simulink model "NeuromuscularModel"  (R2019b)
settings: Solver=ode15s  StartTime=0.0  StopTime=30  MaxStep=.01  RelTol=1e-4  AbsTol=1e-6  EnableMultiTasking=on
values from neighbouring files (symbols this model uses):
  legLengthClr = 0.85    [ControlParams.m]    (also in assignGains.m = Gains(20); assignGainsSagittal.m = GainsSagittal(39))
  LongDelay = 0.020/2    (= 0.01)    [ControlParams.m]
  MidDelay = 0.010/2    (= 0.005)    [ControlParams.m]
  N = {S.name}    [mergeCompareEnergyCosts.m]
  ShortDelay = 0.005/2    (= 0.0025)    [ControlParams.m]
  simbiconGainD = 5*pi/180    (= 0.0872664625997)    [ControlParams.m]    (also in assignGains.m = Gains(21); assignGainsSagittal.m = GainsSagittal(41))
  simbiconGainV = 5*pi/180    (= 0.0872664625997)    [ControlParams.m]    (also in assignGains.m = Gains(22); assignGainsSagittal.m = GainsSagittal(42))
  simbiconLegAngle0 = 70*pi/180    (= 1.2217304764)    [ControlParams.m]    (also in assignGains.m = Gains(23); assignGainsSagittal.m = GainsSagittal(40))
  X = ~cellfun('isempty',strfind(N,'compareEnergyCost'))    [mergeCompareEnergyCosts.m]
undefined symbols (not defined in the file or in its folder): footCenterToCGDist, footInertia, footMass, g, LceOffsetTA, loptGAS, loptTA, lslackGAS, phimaxGASa, phimaxGASk, phirefGASa, phirefGASk, rGASa, rGASk, rhoGASa, rhoGASk, Y, Z
libraries: NeuroMuscularLibrary x85, nesl_utility x23, sm_lib x16, simulink x4, simulink_extras x2
(part 2 of 2)

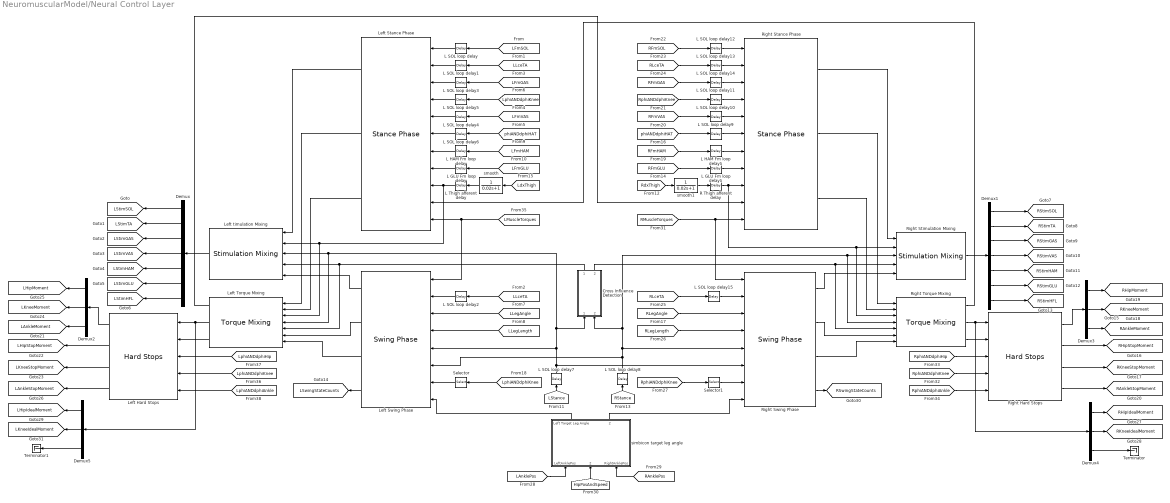
== system NeuromuscularModel/Neural Control Layer ==
  Cross Influence Detection : Subsystem
  Demux : Demux  Outputs=7
  Demux1 : Demux  Outputs=7
  Demux{2..5} (4 alike) : Demux  Outputs=3
  L GLU Fm loop delay : TransportDelay  DelayTime=ShortDelay
  L GLU Fm loop delay1 : TransportDelay  DelayTime=ShortDelay
  L HAM Fm loop delay : TransportDelay  DelayTime=ShortDelay
  L HAM Fm loop delay1 : TransportDelay  DelayTime=ShortDelay
  L SOL loop delay{,1..3,12..15} (8 alike) : TransportDelay  DelayTime=LongDelay
  L SOL loop delay{4..5,7..8,10..11} (6 alike) : TransportDelay  DelayTime=MidDelay
  L SOL loop delay6 : TransportDelay  DelayTime=ShortDelay
  L SOL loop delay9 : TransportDelay  DelayTime=ShortDelay
  L Thigh afferent delay : TransportDelay  DelayTime=ShortDelay
  Left Hard Stops : NeuroMuscularLibrary/Hard Stops  SystemSampleTime=-1  Latency=0  AutoFrameSizeCalculation=off
  Left Stance Phase : NeuroMuscularLibrary/Stance Phase  GainHAM=GainHAM  GainGLU=GainGLU  GainSOL=GainSOL  GainSOLTA=GainSOLTA  GainTA=GainTA  GainGAS=GainGAS  GainVAS=GainVAS  GainKneeOverExt=GainKneeOverExt  PosGainGG=PosGainGG  SpeedGainGG=SpeedGainGG  Kglu=Kglu
  Left Swing Phase : NeuroMuscularLibrary/Swing Phase  GainTA=GainTA  hipPGain=hipPGain  hipDGain=hipDGain  legAngleFilter=legAngleFilter  kneeFlexGain=kneeFlexGain  kneeHoldGain1=kneeHoldGain1  kneeHoldGain2=kneeHoldGain2  kneeStopGain=kneeStopGain  kneeExtendGain=kneeExtendGain  legLengthClr=legLengthClr
  Left Torque Mixing : NeuroMuscularLibrary/Torque Mixing  SystemSampleTime=-1  Latency=0  AutoFrameSizeCalculation=off
  Left timulation Mixing : NeuroMuscularLibrary/Stimulation Mixing  SystemSampleTime=-1  Latency=0  AutoFrameSizeCalculation=off
  R Thigh afferent delay : TransportDelay  DelayTime=ShortDelay
  Right Hard Stops : NeuroMuscularLibrary/Hard Stops  SystemSampleTime=-1  Latency=0  AutoFrameSizeCalculation=off
  Right Stance Phase : NeuroMuscularLibrary/Stance Phase  GainHAM=GainHAM  GainGLU=GainGLU  GainSOL=GainSOL  GainSOLTA=GainSOLTA  GainTA=GainTA  GainGAS=GainGAS  GainVAS=GainVAS  GainKneeOverExt=GainKneeOverExt  PosGainGG=PosGainGG  SpeedGainGG=SpeedGainGG  Kglu=Kglu
  Right Stimulation Mixing : NeuroMuscularLibrary/Stimulation Mixing  SystemSampleTime=-1  Latency=0  AutoFrameSizeCalculation=off
  Right Swing Phase : NeuroMuscularLibrary/Swing Phase  GainTA=GainTA  hipPGain=hipPGain  hipDGain=hipDGain  legAngleFilter=legAngleFilter  kneeFlexGain=kneeFlexGain  kneeHoldGain1=kneeHoldGain1  kneeHoldGain2=kneeHoldGain2  kneeStopGain=kneeStopGain  kneeExtendGain=kneeExtendGain  legLengthClr=legLengthClr
  Right Torque Mixing : NeuroMuscularLibrary/Torque Mixing  SystemSampleTime=-1  Latency=0  AutoFrameSizeCalculation=off
  Selector : Selector  InputPortWidth=2  IndexOptions=Index vector (dialog)  Indices=2  OutputSizes=1
  Selector1 : Selector  InputPortWidth=2  IndexOptions=Index vector (dialog)  Indices=2  OutputSizes=1
  Terminator : Terminator
  Terminator1 : Terminator
  simbicon target leg angle : Subsystem
  smooth : TransferFcn  Denominator=[0.02 1]
  smooth1 : TransferFcn  Denominator=[0.02 1]
  tag scope: LAnkleMoment=global, LAnkleStopMoment=global, LHipIdealMoment=global, LHipMoment=global, LHipStopMoment=global, LKneeIdealMoment=global, LKneeMoment=global, LKneeStopMoment=global, LStimGAS=global, LStimGLU=global, LStimHAM=global, LStimHFL=global, LStimSOL=global, LStimTA=global, LStimVAS=global, LSwingStateCounts=global, RAnkleMoment=global, RAnkleStopMoment=global, RHipIdealMoment=global, RHipMoment=global, RHipStopMoment=global, RKneeIdealMoment=global, RKneeMoment=global, RKneeStopMoment=global, RStimGAS=global, RStimGLU=global, RStimHAM=global, RStimHFL=global, RStimSOL=global, RStimTA=global, RStimVAS=global, RSwingStateCounts=global
  wires:
  [LFmSOL] -> L SOL loop delay/1
  L SOL loop delay/1 -> Left Stance Phase/1
  [LLceTA] -> L SOL loop delay1/1
  L SOL loop delay1/1 -> Left Stance Phase/2
  Demux/1 -> [LStimSOL]
  Demux/2 -> [LStimTA]
  Demux/3 -> [LStimGAS]
  [LFmGAS] -> L SOL loop delay3/1
  L SOL loop delay3/1 -> Left Stance Phase/3
  [LLceTA] -> L SOL loop delay2/1
  L SOL loop delay4/1 -> Left Stance Phase/5
  [LFmVAS] -> L SOL loop delay4/1
  L SOL loop delay5/1 -> Left Stance Phase/4
  [LphiANDdphiKnee] -> L SOL loop delay5/1
  Demux/4 -> [LStimVAS]
  [phiANDdphiHAT] -> L SOL loop delay6/1
  L SOL loop delay6/1 -> Left Stance Phase/6
  Demux/5 -> [LStimHAM]
  Demux/6 -> [LStimGLU]
  Demux/7 -> [LStimHFL]
  [LdxThigh] -> smooth/1
  smooth/1 -> L Thigh afferent delay/1
  [RdxThigh] -> smooth1/1
  smooth1/1 -> R Thigh afferent delay/1
  [LFmHAM] -> L HAM Fm loop delay/1
  [LFmGLU] -> L GLU Fm loop delay/1
  L SOL loop delay7/1 -> Left Torque Mixing/4, Left timulation Mixing/3, Cross Influence Detection/1(LStance), Left Swing Phase/5, Right Swing Phase/6
  [RFmHAM] -> L HAM Fm loop delay1/1
  [RFmGLU] -> L GLU Fm loop delay1/1
  [phiANDdphiHAT] -> L SOL loop delay9/1
  L SOL loop delay9/1 -> Right Stance Phase/6
  Demux1/1 -> [RStimSOL]
  Demux1/2 -> [RStimTA]
  Demux1/4 -> [RStimVAS]
  Demux1/5 -> [RStimHAM]
  Demux1/7 -> [RStimHFL]
  Demux1/3 -> [RStimGAS]
  [LStance] -> L SOL loop delay7/1
  [RStance] -> L SOL loop delay8/1
  [RFmVAS] -> L SOL loop delay10/1
  [RphiANDdphiKnee] -> L SOL loop delay11/1
  L SOL loop delay10/1 -> Right Stance Phase/5
  L SOL loop delay11/1 -> Right Stance Phase/4
  L SOL loop delay12/1 -> Right Stance Phase/1
  [RFmSOL] -> L SOL loop delay12/1
  [RLceTA] -> L SOL loop delay13/1
  L SOL loop delay13/1 -> Right Stance Phase/2
  [RFmGAS] -> L SOL loop delay14/1
  L SOL loop delay14/1 -> Right Stance Phase/3
  [RLceTA] -> L SOL loop delay15/1
  Demux1/6 -> [RStimGLU]
  L Thigh afferent delay/1 -> Left Torque Mixing/3, Left timulation Mixing/2, Left Stance Phase/9
  L HAM Fm loop delay/1 -> Left Stance Phase/7
  L GLU Fm loop delay/1 -> Left Stance Phase/8
  R Thigh afferent delay/1 -> Right Stimulation Mixing/2, Right Torque Mixing/3, Right Stance Phase/9
  L HAM Fm loop delay1/1 -> Right Stance Phase/7
  L GLU Fm loop delay1/1 -> Right Stance Phase/8
  L SOL loop delay15/1 -> Right Swing Phase/2
  L SOL loop delay2/1 -> Left Swing Phase/2
  Right Stimulation Mixing/1 -> Demux1/1
  Right Stance Phase/1 -> Right Stimulation Mixing/1
  L SOL loop delay8/1 -> Right Stimulation Mixing/3, Right Torque Mixing/4, Cross Influence Detection/2(RStance), Right Swing Phase/5, Left Swing Phase/6
  Cross Influence Detection/2(LeftLeading) -> Right Stimulation Mixing/4, Right Torque Mixing/5
  Left timulation Mixing/1 -> Demux/1
  Left Stance Phase/1 -> Left timulation Mixing/1
  Cross Influence Detection/1(RightLeading) -> Left Torque Mixing/5, Left timulation Mixing/4
  Demux3/1 -> [RHipMoment]
  Demux3/2 -> [RKneeMoment]
  [LLegAngle] -> Left Swing Phase/3
  [LLegLength] -> Left Swing Phase/4
  [RLegAngle] -> Right Swing Phase/3
  [RLegLength] -> Right Swing Phase/4
  [RphiANDdphiKnee] -> Selector1/1
  Selector1/1 -> Right Swing Phase/7
  [LAnklePos] -> simbicon target leg angle/1(LeftAnklePos)
  [RAnklePos] -> simbicon target leg angle/3(RightAnklePos)
  Right Swing Phase/1 -> Right Stimulation Mixing/5
  [LphiANDdphiKnee] -> Selector/1
  Selector/1 -> Left Swing Phase/7
  Left Swing Phase/1 -> Left timulation Mixing/5
  [HipPosAndSpeed] -> simbicon target leg angle/2(HIPposAndSpeed)
  simbicon target leg angle/2(Right Target Leg Angle) -> Right Swing Phase/8
  simbicon target leg angle/1(Left Target Leg Angle) -> Left Swing Phase/8
  Right Swing Phase/4 -> [RSwingStateCounts]
  Left Swing Phase/4 -> [LSwingStateCounts]
  Demux3/3 -> [RAnkleMoment]
  [RphiANDdphiKnee] -> Right Hard Stops/4
  [RphiANDdphiHip] -> Right Hard Stops/3
  [RphiANDdphiAnkle] -> Right Hard Stops/5
  Right Hard Stops/2 -> [RHipStopMoment]
  Right Hard Stops/3 -> [RKneeStopMoment]
  Right Hard Stops/4 -> [RAnkleStopMoment]
  [LMuscleTorques] -> Left Swing Phase/1, Left Stance Phase/11
  Demux2/1 -> [LHipMoment]
  Demux2/3 -> [LAnkleMoment]
  Left Hard Stops/1 -> Demux2/1
  [LphiANDdphiKnee] -> Left Hard Stops/4
  [LphiANDdphiHip] -> Left Hard Stops/3
  Left Hard Stops/2 -> [LHipStopMoment]
  Left Hard Stops/3 -> [LKneeStopMoment]
  Left Hard Stops/4 -> [LAnkleStopMoment]
  Left Stance Phase/2 -> Left Torque Mixing/1
  Demux2/2 -> [LKneeMoment]
  Right Torque Mixing/2 -> Demux4/1, Right Hard Stops/1
  Right Hard Stops/1 -> Demux3/1
  [RMuscleTorques] -> Right Swing Phase/1, Right Stance Phase/11
  Demux4/1 -> [RHipIdealMoment]
  Demux4/2 -> [RKneeIdealMoment]
  Demux4/3 -> Terminator/1
  Right Swing Phase/3 -> Right Torque Mixing/7
  Right Swing Phase/2 -> Right Torque Mixing/6
  Right Stance Phase/3 -> Right Torque Mixing/2
  Right Stance Phase/2 -> Right Torque Mixing/1
  Right Torque Mixing/3 -> Right Hard Stops/2
  Right Torque Mixing/1 -> Left Stance Phase/10
  [LphiANDdphiAnkle] -> Left Hard Stops/5
  Left Torque Mixing/2 -> Demux5/1, Left Hard Stops/1
  Left Torque Mixing/3 -> Left Hard Stops/2
  Left Torque Mixing/1 -> Right Stance Phase/10
  Left Stance Phase/3 -> Left Torque Mixing/2
  Left Swing Phase/2 -> Left Torque Mixing/6
  Left Swing Phase/3 -> Left Torque Mixing/7
  Demux5/1 -> [LHipIdealMoment]
  Demux5/2 -> [LKneeIdealMoment]
  Demux5/3 -> Terminator1/1

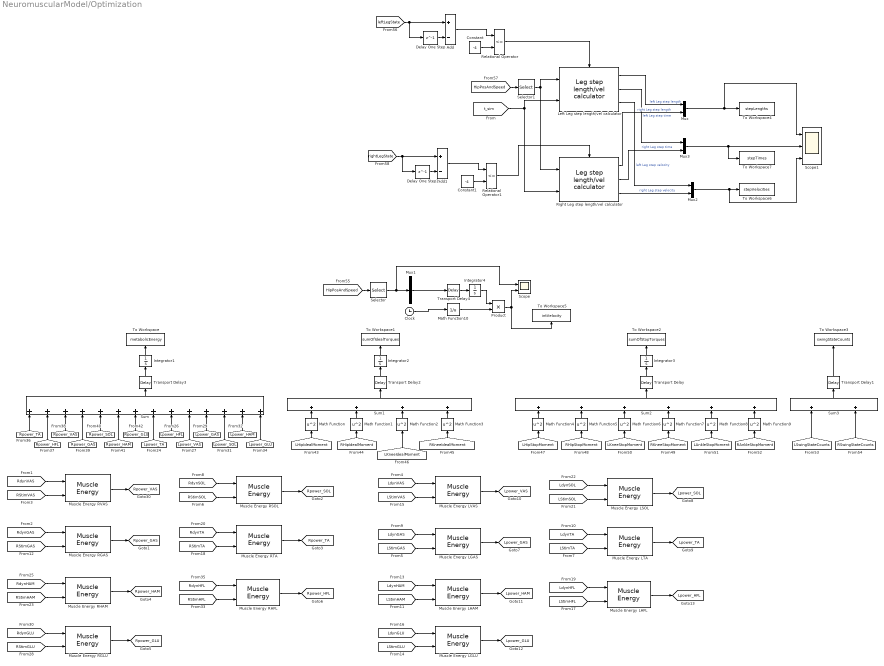
== system NeuromuscularModel/Optimization ==
  Add : Sum  Inputs=+-
  Add1 : Sum  Inputs=+-
  Clock : Clock
      settings: Decimation=1000
  Constant : Constant  Value=-4
  Constant1 : Constant  Value=-4
  Delay One Step : Delay  DelayLength=1
  Delay One Step1 : Delay  DelayLength=1
  Integrator{1..4} (4 alike) : Integrator
  Left Leg step length/vel calculator : NeuroMuscularLibrary/Leg step length//vel calculator  SystemSampleTime=-1  Latency=0  AutoFrameSizeCalculation=off
  Math Function{,1..9} (10 alike) : Math  Operator=square  SaturateOnIntegerOverflow=on
  Math Function10 : Math  Operator=reciprocal  SignedPower=off  SaturateOnIntegerOverflow=on
  Muscle Energy LGAS : NeuroMuscularLibrary/Muscle Energy  lopt=loptGAS  FT=FT_GAS  Fmax=FmaxGAS
  Muscle Energy LGLU : NeuroMuscularLibrary/Muscle Energy  lopt=loptGLU  FT=FT_GLU  Fmax=FmaxGLU
  Muscle Energy LHAM : NeuroMuscularLibrary/Muscle Energy  lopt=loptHAM  FT=FT_HAM  Fmax=FmaxHAM
  Muscle Energy LHFL : NeuroMuscularLibrary/Muscle Energy  lopt=loptHFL  FT=FT_HFL  Fmax=FmaxHFL
  Muscle Energy LSOL : NeuroMuscularLibrary/Muscle Energy  lopt=loptSOL  FT=FT_SOL  Fmax=FmaxSOL
  Muscle Energy LTA : NeuroMuscularLibrary/Muscle Energy  lopt=loptTA  FT=FT_TA  Fmax=FmaxTA
  Muscle Energy LVAS : NeuroMuscularLibrary/Muscle Energy  lopt=loptVAS  FT=FT_VAS  Fmax=FmaxVAS
  Muscle Energy RGAS : NeuroMuscularLibrary/Muscle Energy  lopt=loptGAS  FT=FT_GAS  Fmax=FmaxGAS
  Muscle Energy RGLU : NeuroMuscularLibrary/Muscle Energy  lopt=loptGLU  FT=FT_GLU  Fmax=FmaxGLU
  Muscle Energy RHAM : NeuroMuscularLibrary/Muscle Energy  lopt=loptHAM  FT=FT_HAM  Fmax=FmaxHAM
  Muscle Energy RHFL : NeuroMuscularLibrary/Muscle Energy  lopt=loptHFL  FT=FT_HFL  Fmax=FmaxHFL
  Muscle Energy RSOL : NeuroMuscularLibrary/Muscle Energy  lopt=loptSOL  FT=FT_SOL  Fmax=FmaxSOL
  Muscle Energy RTA : NeuroMuscularLibrary/Muscle Energy  lopt=loptTA  FT=FT_TA  Fmax=FmaxTA
  Muscle Energy RVAS : NeuroMuscularLibrary/Muscle Energy  lopt=loptVAS  FT=FT_VAS  Fmax=FmaxVAS
  Mux : Mux  Inputs=2
  Mux1 : Mux  Inputs=1
  Mux2 : Mux  Inputs=2
  Mux3 : Mux  Inputs=2
  Product : Product
  Relational Operator : RelationalOperator  Operator=<=  OutDataTypeStr=boolean  RndMeth=Simplest
  Relational Operator1 : RelationalOperator  Operator=<=  OutDataTypeStr=boolean  RndMeth=Simplest
  Right Leg step length/vel calculator : NeuroMuscularLibrary/Leg step length//vel calculator  SystemSampleTime=-1  Latency=0  AutoFrameSizeCalculation=off
  Scope : Scope  NumInputPorts=2
  Scope1 : Scope  NumInputPorts=3
  Selector : Selector  InputPortWidth=3  IndexOptions=Index vector (dialog)  Indices=[3]  OutputSizes=1
  Selector1 : Selector  InputPortWidth=3  IndexOptions=Index vector (dialog)  Indices=[1]  OutputSizes=1
  Sum : Sum  Inputs=++++++++++++++
  Sum1 : Sum  Inputs=++++
  Sum2 : Sum  Inputs=++++++
  Sum3 : Sum
  To Workspace : ToWorkspace  VariableName=metabolicEnergy  SampleTime=-1
      settings: MaxDataPoints=1
  To Workspace1 : ToWorkspace  VariableName=sumOfIdealTorques  SampleTime=-1
      settings: MaxDataPoints=1
  To Workspace2 : ToWorkspace  VariableName=sumOfStopTorques  SampleTime=-1
      settings: MaxDataPoints=1
  To Workspace3 : ToWorkspace  VariableName=swingStateCounts  SampleTime=-1
      settings: MaxDataPoints=1
  To Workspace4 : ToWorkspace  VariableName=stepLengths  SampleTime=-1
  To Workspace5 : ToWorkspace  VariableName=intVelocity  SampleTime=-1
      settings: MaxDataPoints=1
  To Workspace6 : ToWorkspace  VariableName=stepVelocities  SampleTime=-1
  To Workspace7 : ToWorkspace  VariableName=stepTimes  SaveFormat=Structure With Time  SampleTime=-1
  Transport Delay{,1..3} (4 alike) : TransportDelay  DelayTime=3  BufferSize=24576
  Transport Delay4 : TransportDelay  DelayTime=0.2  BufferSize=24576
  tag scope: Lpower_GAS=global, Lpower_GLU=global, Lpower_HAM=global, Lpower_HFL=global, Lpower_SOL=global, Lpower_TA=global, Lpower_VAS=global, Rpower_GAS=global, Rpower_GLU=global, Rpower_HAM=global, Rpower_HFL=global, Rpower_SOL=global, Rpower_TA=global, Rpower_VAS=global
  wires:
  [RdynSOL] -> Muscle Energy RSOL/1
  [RStimSOL] -> Muscle Energy RSOL/2
  [RStimVAS] -> Muscle Energy RVAS/2
  [RStimGAS] -> Muscle Energy RGAS/2
  Muscle Energy RVAS/1 -> [Rpower_VAS]
  Muscle Energy RGAS/1 -> [Rpower_GAS]
  Muscle Energy RSOL/1 -> [Rpower_SOL]
  Muscle Energy RTA/1 -> [Rpower_TA]
  [RdynTA] -> Muscle Energy RTA/1
  [RStimTA] -> Muscle Energy RTA/2
  [RdynHAM] -> Muscle Energy RHAM/1
  [RStimHAM] -> Muscle Energy RHAM/2
  [RdynGLU] -> Muscle Energy RGLU/1
  [RStimGLU] -> Muscle Energy RGLU/2
  [RdynHFL] -> Muscle Energy RHFL/1
  [RStimHFL] -> Muscle Energy RHFL/2
  Muscle Energy RHAM/1 -> [Rpower_HAM]
  Muscle Energy RGLU/1 -> [Rpower_GLU]
  Muscle Energy RHFL/1 -> [Rpower_HFL]
  [Rpower_TA] -> Sum/1
  [Rpower_GLU] -> Sum/7
  [Rpower_HAM] -> Sum/6
  [Rpower_SOL] -> Sum/5
  [Rpower_GAS] -> Sum/4
  [Rpower_VAS] -> Sum/3
  [Rpower_HFL] -> Sum/2
  [RdynGAS] -> Muscle Energy RGAS/1
  [RdynVAS] -> Muscle Energy RVAS/1
  [LdynSOL] -> Muscle Energy LSOL/1
  [LStimSOL] -> Muscle Energy LSOL/2
  [LStimVAS] -> Muscle Energy LVAS/2
  [LStimGAS] -> Muscle Energy LGAS/2
  Muscle Energy LVAS/1 -> [Lpower_VAS]
  Muscle Energy LGAS/1 -> [Lpower_GAS]
  Muscle Energy LSOL/1 -> [Lpower_SOL]
  Muscle Energy LTA/1 -> [Lpower_TA]
  [LdynTA] -> Muscle Energy LTA/1
  [LStimTA] -> Muscle Energy LTA/2
  [LdynHAM] -> Muscle Energy LHAM/1
  [LStimHAM] -> Muscle Energy LHAM/2
  [LdynGLU] -> Muscle Energy LGLU/1
  [LStimGLU] -> Muscle Energy LGLU/2
  [LdynHFL] -> Muscle Energy LHFL/1
  [LStimHFL] -> Muscle Energy LHFL/2
  Muscle Energy LHAM/1 -> [Lpower_HAM]
  Muscle Energy LGLU/1 -> [Lpower_GLU]
  Muscle Energy LHFL/1 -> [Lpower_HFL]
  [LdynGAS] -> Muscle Energy LGAS/1
  [LdynVAS] -> Muscle Energy LVAS/1
  [Lpower_TA] -> Sum/8
  [Lpower_GLU] -> Sum/14
  [Lpower_HAM] -> Sum/13
  [Lpower_SOL] -> Sum/12
  [Lpower_GAS] -> Sum/11
  [Lpower_VAS] -> Sum/10
  [Lpower_HFL] -> Sum/9
  Integrator1/1 -> To Workspace/1
  Sum/1 -> Transport Delay3/1
  Integrator2/1 -> To Workspace1/1
  Sum1/1 -> Transport Delay2/1
  Math Function/1 -> Sum1/1
  [LHipIdealMoment] -> Math Function/1
  Math Function1/1 -> Sum1/2
  [RHipIdealMoment] -> Math Function1/1
  Math Function2/1 -> Sum1/3
  Math Function3/1 -> Sum1/4
  [LKneeIdealMoment] -> Math Function2/1
  [RKneeIdealMoment] -> Math Function3/1
  Integrator3/1 -> To Workspace2/1
  Math Function4/1 -> Sum2/1
  [LHipStopMoment] -> Math Function4/1
  Math Function5/1 -> Sum2/2
  [RHipStopMoment] -> Math Function5/1
  Math Function6/1 -> Sum2/3
  Math Function7/1 -> Sum2/4
  [LKneeStopMoment] -> Math Function6/1
  [RKneeStopMoment] -> Math Function7/1
  [LAnkleStopMoment] -> Math Function8/1
  Math Function8/1 -> Sum2/5
  [RAnkleStopMoment] -> Math Function9/1
  Math Function9/1 -> Sum2/6
  Transport Delay/1 -> Integrator3/1
  Sum2/1 -> Transport Delay/1
  Sum3/1 -> Transport Delay1/1
  Transport Delay1/1 -> To Workspace3/1
  [LSwingStateCounts] -> Sum3/1
  [RSwingStateCounts] -> Sum3/2
  Transport Delay2/1 -> Integrator2/1
  Transport Delay3/1 -> Integrator1/1
  Selector/1 -> Scope/1, Mux1/1
  [HipPosAndSpeed] -> Selector/1
  Mux1/1 -> Transport Delay4/1
  Transport Delay4/1 -> Integrator4/1
  Integrator4/1 -> Product/1
  Clock/1 -> Math Function10/1
  Math Function10/1 -> Product/2
  Product/1 -> To Workspace5/1, Scope/2
  [leftLegState] -> Add/1, Delay One Step/1
  Delay One Step/1 -> Add/2
  Add/1 -> Relational Operator/1
  [HipPosAndSpeed] -> Selector1/1
  Constant/1 -> Relational Operator/2
  Selector1/1 -> Right Leg step length/vel calculator/1, Left Leg step length/vel calculator/1
  Relational Operator/1 -> Left Leg step length/vel calculator/Enable
  Left Leg step length/vel calculator/1 -> Mux/1  "left Leg step length"
  Constant1/1 -> Relational Operator1/2
  Add1/1 -> Relational Operator1/1
  Delay One Step1/1 -> Add1/2
  [rightLegState] -> Delay One Step1/1, Add1/1
  Relational Operator1/1 -> Right Leg step length/vel calculator/Enable
  Right Leg step length/vel calculator/1 -> Mux/2  "right Leg step length"
  Mux/1 -> To Workspace4/1, Scope1/1
  [t_sim] -> Right Leg step length/vel calculator/2, Left Leg step length/vel calculator/2
  Mux2/1 -> To Workspace6/1, Scope1/3
  Left Leg step length/vel calculator/3 -> Mux2/1  "left Leg step velocity"
  Right Leg step length/vel calculator/3 -> Mux2/2  "right Leg step velocity"
  Mux3/1 -> Scope1/2, To Workspace7/1
  Left Leg step length/vel calculator/2 -> Mux3/1  "left Leg step time"
  Right Leg step length/vel calculator/2 -> Mux3/2  "right Leg step time"

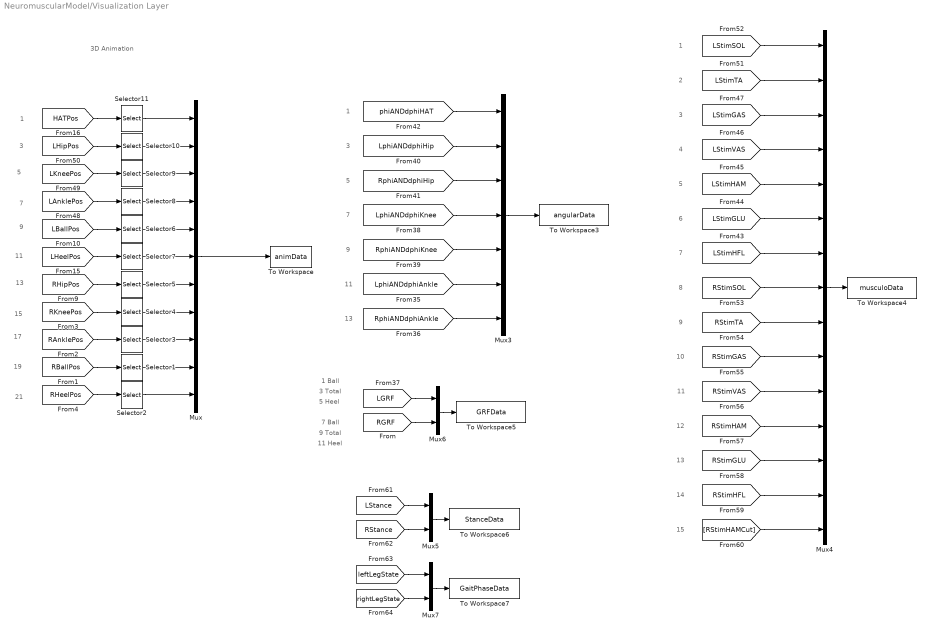
== system NeuromuscularModel/Visualization Layer ==
  note: 21
  note: 19
  note: 17
  note: 15
  note: 13
  note: 11
  note: 9
  note: 7
  note: 5
  note: 3
  note: 1
  note: 3D Animation
  note: 1
  note: 8
  note: 13
  note: 3
  note: 1
  note: 5
  note: 10
  note: 4
  note: 6
  note: 3
  note: 5
  note: 7
  note: 9
  note: 9
  note: 11
  note: 2
  note: 7
  note: 11
  note: 12
  note: 15
  note: 9 Total
  note: 1 Ball
  note: 5 Heel
  note: 14
  note: 11 Heel
  note: 3 Total
  note: 13
  note: 7 Ball
  Mux : Mux  Inputs=11
  Mux3 : Mux  Inputs=7
  Mux4 : Mux  Inputs=15
  Mux5 : Mux  Inputs=2
  Mux6 : Mux  Inputs=2
  Mux7 : Mux  Inputs=2
  Selector{1..11} (11 alike) : Selector  InputPortWidth=3  IndexOptions=Index vector (dialog)  Indices=[1 3]  OutputSizes=1
  To Workspace : ToWorkspace  VariableName=animData  SaveFormat=Structure With Time  SampleTime=1/30
  To Workspace3 : ToWorkspace  VariableName=angularData  SaveFormat=Structure With Time  SampleTime=1/30
  To Workspace4 : ToWorkspace  VariableName=musculoData  SaveFormat=Structure With Time  SampleTime=1/30
  To Workspace5 : ToWorkspace  VariableName=GRFData  SaveFormat=Structure With Time  SampleTime=1/30
  To Workspace6 : ToWorkspace  VariableName=StanceData  SaveFormat=Structure With Time  SampleTime=1/30
  To Workspace7 : ToWorkspace  VariableName=GaitPhaseData  SaveFormat=Structure With Time  SampleTime=1/30
  wires:
  [RAnklePos] -> Selector3/1
  [RKneePos] -> Selector4/1
  [RHipPos] -> Selector5/1
  [HATPos] -> Selector11/1
  [LHeelPos] -> Selector7/1
  [LBallPos] -> Selector6/1
  [LAnklePos] -> Selector8/1
  [LKneePos] -> Selector9/1
  [LHipPos] -> Selector10/1
  Selector11/1 -> Mux/1
  Selector3/1 -> Mux/9
  Selector4/1 -> Mux/8
  Selector5/1 -> Mux/7
  Selector7/1 -> Mux/6
  Selector6/1 -> Mux/5
  Selector8/1 -> Mux/4
  Selector9/1 -> Mux/3
  Selector10/1 -> Mux/2
  Mux/1 -> To Workspace/1
  [RHeelPos] -> Selector2/1
  [RBallPos] -> Selector1/1
  Selector2/1 -> Mux/11
  Selector1/1 -> Mux/10
  [LStance] -> Mux5/1
  [LStimGLU] -> Mux4/6
  Mux4/1 -> To Workspace4/1
  [RphiANDdphiAnkle] -> Mux3/7
  Mux5/1 -> To Workspace6/1
  Mux6/1 -> To Workspace5/1
  [RStimGLU] -> Mux4/13
  [RGRF] -> Mux6/2
  [phiANDdphiHAT] -> Mux3/1
  [RStimTA] -> Mux4/9
  Mux3/1 -> To Workspace3/1
  [LphiANDdphiAnkle] -> Mux3/6
  [RStimVAS] -> Mux4/11
  [LphiANDdphiKnee] -> Mux3/4
  [RStimHAM] -> Mux4/12
  [RStimHAMCut] -> Mux4/15
  [LGRF] -> Mux6/1
  [RStimHFL] -> Mux4/14
  [LphiANDdphiHip] -> Mux3/2
  [RStimSOL] -> Mux4/8
  [RphiANDdphiKnee] -> Mux3/5
  [LStimGAS] -> Mux4/3
  [LStimSOL] -> Mux4/1
  [LStimHAM] -> Mux4/5
  [RStimGAS] -> Mux4/10
  [LStimHFL] -> Mux4/7
  [LStimTA] -> Mux4/2
  [RStance] -> Mux5/2
  [RphiANDdphiHip] -> Mux3/3
  [LStimVAS] -> Mux4/4
  [rightLegState] -> Mux7/2
  Mux7/1 -> To Workspace7/1
  [leftLegState] -> Mux7/1

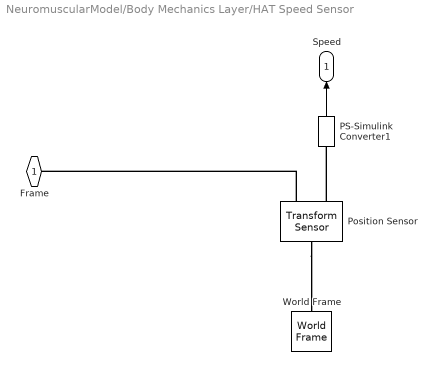
== system NeuromuscularModel/Body Mechanics Layer/HAT Speed Sensor ==
  PS-Simulink Converter1 : nesl_utility/PS-Simulink Converter  PhysicalDomain=network_engine_domain  SubClassName=ps_output  LeftPortType=input  RightPortType=output  PseudoPeriodic=off  Frequencies=[]  Unit=m/s  AffineConversion=off
  Position Sensor : sm_lib/Frames and Transforms/Transform Sensor  MeasurementFrame=World  SenseAngle=off  SenseAxis=off  SenseAngle1=off  SenseAngle2=off  SenseAngle3=off  SenseQ=off  SenseR=off  SenseOmegaX=off  SenseOmegaY=off  SenseOmegaZ=off  SenseOmega1=off  SenseOmega2=off  SenseOmega3=off  SenseQDot=off  SenseRDot=off  SenseAlphaX=off  SenseAlphaY=off  SenseAlphaZ=off  SenseAlpha1=off  SenseAlpha2=off  SenseAlpha3=off  SenseQDDot=off  SenseRDDot=off  SenseX=off  SenseY=off  SenseZ=off  SenseRad=off  SenseAzim=off  SenseDist=off  SenseInc=off  SenseXDot=on  SenseYDot=off  SenseZDot=off  SenseRadDot=off  SenseAzimDot=off  SenseDistDot=off  SenseIncDot=off  SenseXDDot=off  SenseYDDot=off  SenseZDDot=off  SenseRadDDot=off  SenseAzimDDot=off  SenseDistDDot=off  SenseIncDDot=off
  World Frame : sm_lib/Frames and Transforms/World Frame
  Frame : PMIOPort  Side=Left
  Speed : Outport
  wires:
  PS-Simulink Converter1/1 -> Speed/1
  connections:
  Position Sensor/LConn1 -- World Frame/RConn1
  Position Sensor/RConn1 -- Frame/RConn1
  Position Sensor/RConn2 -- PS-Simulink Converter1/LConn1

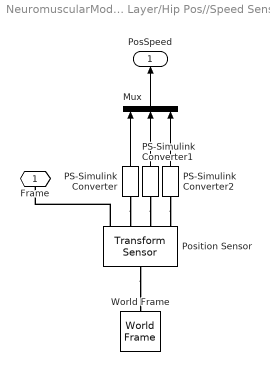
== system NeuromuscularModel/Body Mechanics Layer/Hip Pos//Speed Sensor ==
  Mux : Mux  Inputs=3
  PS-Simulink Converter : nesl_utility/PS-Simulink Converter  PhysicalDomain=network_engine_domain  SubClassName=ps_output  LeftPortType=input  RightPortType=output  PseudoPeriodic=off  Frequencies=[]  Unit=m  AffineConversion=off
  PS-Simulink Converter1 : nesl_utility/PS-Simulink Converter  PhysicalDomain=network_engine_domain  SubClassName=ps_output  LeftPortType=input  RightPortType=output  PseudoPeriodic=off  Frequencies=[]  Unit=m  AffineConversion=off
  PS-Simulink Converter2 : nesl_utility/PS-Simulink Converter  PhysicalDomain=network_engine_domain  SubClassName=ps_output  LeftPortType=input  RightPortType=output  PseudoPeriodic=off  Frequencies=[]  Unit=m/s  AffineConversion=off
  Position Sensor : sm_lib/Frames and Transforms/Transform Sensor  MeasurementFrame=World  SenseAngle=off  SenseAxis=off  SenseAngle1=off  SenseAngle2=off  SenseAngle3=off  SenseQ=off  SenseR=off  SenseOmegaX=off  SenseOmegaY=off  SenseOmegaZ=off  SenseOmega1=off  SenseOmega2=off  SenseOmega3=off  SenseQDot=off  SenseRDot=off  SenseAlphaX=off  SenseAlphaY=off  SenseAlphaZ=off  SenseAlpha1=off  SenseAlpha2=off  SenseAlpha3=off  SenseQDDot=off  SenseRDDot=off  SenseX=on  SenseY=off  SenseZ=on  SenseRad=off  SenseAzim=off  SenseDist=off  SenseInc=off  SenseXDot=on  SenseYDot=off  SenseZDot=off  SenseRadDot=off  SenseAzimDot=off  SenseDistDot=off  SenseIncDot=off  SenseXDDot=off  SenseYDDot=off  SenseZDDot=off  SenseRadDDot=off  SenseAzimDDot=off  SenseDistDDot=off  SenseIncDDot=off
  World Frame : sm_lib/Frames and Transforms/World Frame
  Frame : PMIOPort  Side=Left
  PosSpeed : Outport
  wires:
  Mux/1 -> PosSpeed/1
  PS-Simulink Converter/1 -> Mux/1
  PS-Simulink Converter1/1 -> Mux/2
  PS-Simulink Converter2/1 -> Mux/3
  connections:
  Position Sensor/LConn1 -- World Frame/RConn1
  Position Sensor/RConn1 -- Frame/RConn1
  PS-Simulink Converter/LConn1 -- Position Sensor/RConn2
  PS-Simulink Converter1/LConn1 -- Position Sensor/RConn3
  PS-Simulink Converter2/LConn1 -- Position Sensor/RConn4

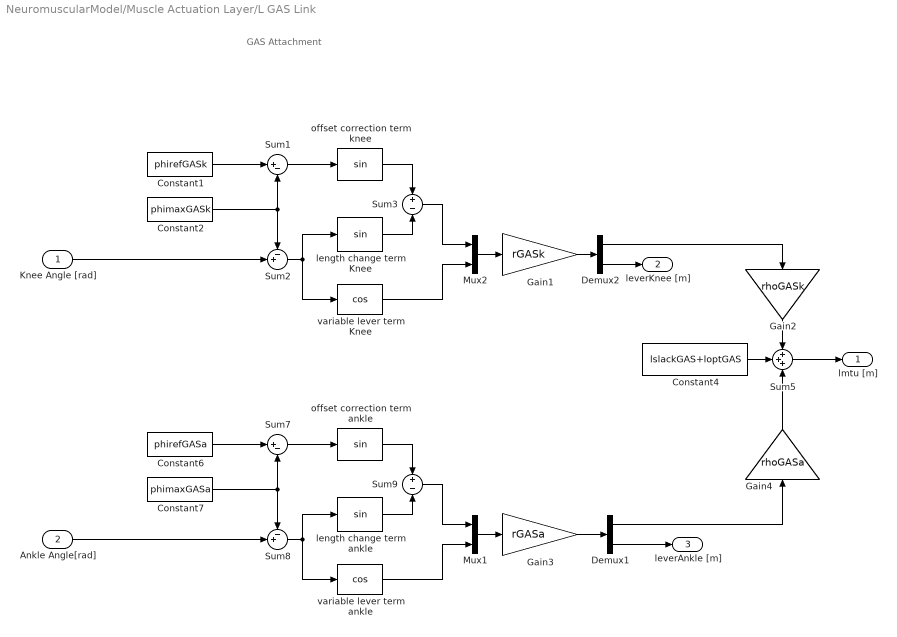
== system NeuromuscularModel/Muscle Actuation Layer/L GAS Link ==
  note: GAS Attachment
  Knee Angle [rad] : Inport
  Ankle Angle[rad] : Inport  Port=2
  Constant1 : Constant  Value=phirefGASk
  Constant2 : Constant  Value=phimaxGASk
  Constant4 : Constant  Value=lslackGAS+loptGAS
  Constant6 : Constant  Value=phirefGASa
  Constant7 : Constant  Value=phimaxGASa
  Demux1 : Demux  Outputs=2
  Demux2 : Demux  Outputs=2
  Gain1 : Gain  Gain=rGASk
  Gain2 : Gain  Gain=rhoGASk
  Gain3 : Gain  Gain=rGASa
  Gain4 : Gain  Gain=rhoGASa
  Mux1 : Mux  Inputs=2
  Mux2 : Mux  Inputs=2
  Sum1 : Sum  Inputs=|+-
  Sum2 : Sum  Inputs=-+|
  Sum3 : Sum  Inputs=+-
  Sum5 : Sum  Inputs=+++
  Sum7 : Sum  Inputs=|+-
  Sum8 : Sum  Inputs=-+|
  Sum9 : Sum  Inputs=+-
  length change term Knee : Trigonometry
  length change term ankle : Trigonometry
  offset correction term ankle : Trigonometry
  offset correction term knee : Trigonometry
  variable lever term Knee : Trigonometry  Operator=cos
  variable lever term ankle : Trigonometry  Operator=cos
  lmtu [m] : Outport
  leverKnee [m] : Outport  Port=2
  leverAnkle [m] : Outport  Port=3
  wires:
  Ankle Angle[rad]/1 -> Sum8/2
  Sum5/1 -> lmtu [m]/1
  variable lever term ankle/1 -> Mux1/2
  Demux1/2 -> leverAnkle [m]/1
  Sum8/1 -> variable lever term ankle/1, length change term ankle/1
  Constant7/1 -> Sum8/1, Sum7/2
  Sum7/1 -> offset correction term ankle/1
  Constant6/1 -> Sum7/1
  length change term ankle/1 -> Sum9/2
  offset correction term ankle/1 -> Sum9/1
  Sum9/1 -> Mux1/1
  Constant4/1 -> Sum5/2
  Mux1/1 -> Gain3/1
  Gain3/1 -> Demux1/1
  Demux1/1 -> Gain4/1
  Gain4/1 -> Sum5/3
  Knee Angle [rad]/1 -> Sum2/2
  variable lever term Knee/1 -> Mux2/2
  Sum2/1 -> variable lever term Knee/1, length change term Knee/1
  Constant2/1 -> Sum2/1, Sum1/2
  Sum1/1 -> offset correction term knee/1
  Constant1/1 -> Sum1/1
  length change term Knee/1 -> Sum3/2
  offset correction term knee/1 -> Sum3/1
  Sum3/1 -> Mux2/1
  Mux2/1 -> Gain1/1
  Gain1/1 -> Demux2/1
  Demux2/2 -> leverKnee [m]/1
  Demux2/1 -> Gain2/1
  Gain2/1 -> Sum5/1

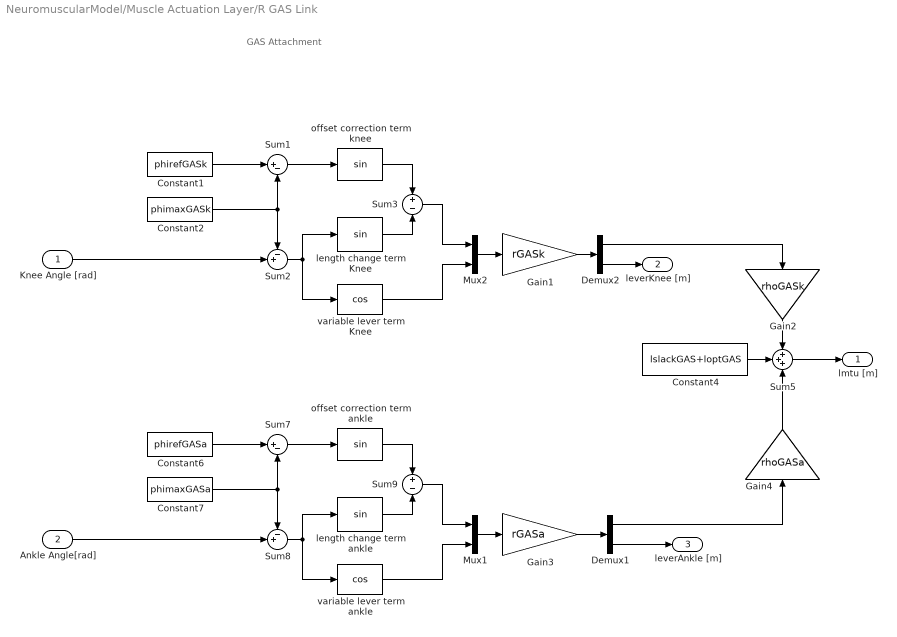
== system NeuromuscularModel/Muscle Actuation Layer/R GAS Link ==
  note: GAS Attachment
  Knee Angle [rad] : Inport
  Ankle Angle[rad] : Inport  Port=2
  Constant1 : Constant  Value=phirefGASk
  Constant2 : Constant  Value=phimaxGASk
  Constant4 : Constant  Value=lslackGAS+loptGAS
  Constant6 : Constant  Value=phirefGASa
  Constant7 : Constant  Value=phimaxGASa
  Demux1 : Demux  Outputs=2
  Demux2 : Demux  Outputs=2
  Gain1 : Gain  Gain=rGASk
  Gain2 : Gain  Gain=rhoGASk
  Gain3 : Gain  Gain=rGASa
  Gain4 : Gain  Gain=rhoGASa
  Mux1 : Mux  Inputs=2
  Mux2 : Mux  Inputs=2
  Sum1 : Sum  Inputs=|+-
  Sum2 : Sum  Inputs=-+|
  Sum3 : Sum  Inputs=+-
  Sum5 : Sum  Inputs=+++
  Sum7 : Sum  Inputs=|+-
  Sum8 : Sum  Inputs=-+|
  Sum9 : Sum  Inputs=+-
  length change term Knee : Trigonometry
  length change term ankle : Trigonometry
  offset correction term ankle : Trigonometry
  offset correction term knee : Trigonometry
  variable lever term Knee : Trigonometry  Operator=cos
  variable lever term ankle : Trigonometry  Operator=cos
  lmtu [m] : Outport
  leverKnee [m] : Outport  Port=2
  leverAnkle [m] : Outport  Port=3
  wires:
  Ankle Angle[rad]/1 -> Sum8/2
  Sum5/1 -> lmtu [m]/1
  variable lever term ankle/1 -> Mux1/2
  Demux1/2 -> leverAnkle [m]/1
  Sum8/1 -> variable lever term ankle/1, length change term ankle/1
  Constant7/1 -> Sum8/1, Sum7/2
  Sum7/1 -> offset correction term ankle/1
  Constant6/1 -> Sum7/1
  length change term ankle/1 -> Sum9/2
  offset correction term ankle/1 -> Sum9/1
  Sum9/1 -> Mux1/1
  Constant4/1 -> Sum5/2
  Mux1/1 -> Gain3/1
  Gain3/1 -> Demux1/1
  Demux1/1 -> Gain4/1
  Gain4/1 -> Sum5/3
  Knee Angle [rad]/1 -> Sum2/2
  variable lever term Knee/1 -> Mux2/2
  Sum2/1 -> variable lever term Knee/1, length change term Knee/1
  Constant2/1 -> Sum2/1, Sum1/2
  Sum1/1 -> offset correction term knee/1
  Constant1/1 -> Sum1/1
  length change term Knee/1 -> Sum3/2
  offset correction term knee/1 -> Sum3/1
  Sum3/1 -> Mux2/1
  Mux2/1 -> Gain1/1
  Gain1/1 -> Demux2/1
  Demux2/2 -> leverKnee [m]/1
  Demux2/1 -> Gain2/1
  Gain2/1 -> Sum5/1

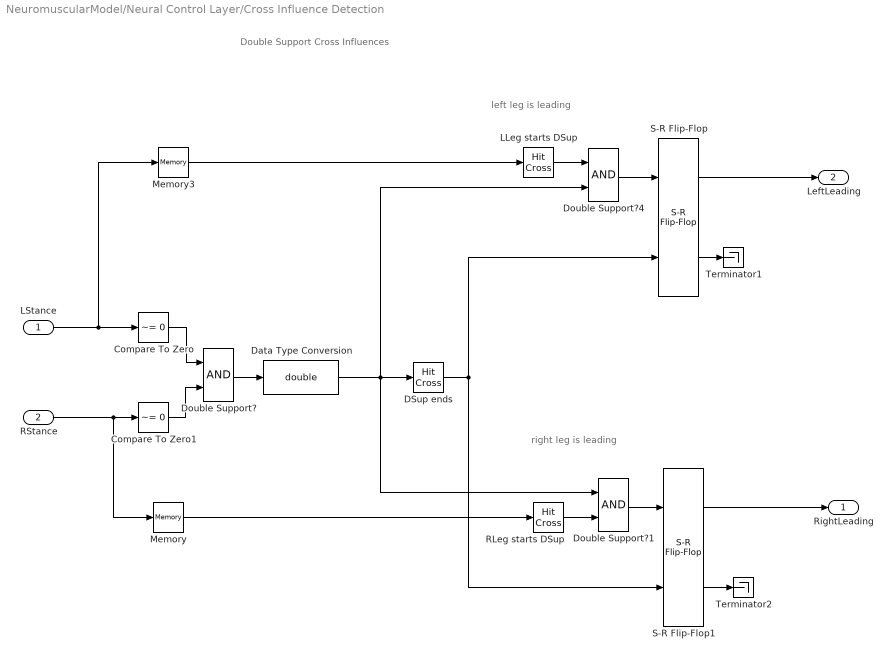
== system NeuromuscularModel/Neural Control Layer/Cross Influence Detection ==
  note: right leg is leading
  note: left leg is leading
  note: Double Support Cross Influences
  LStance : Inport
  RStance : Inport  Port=2
  Compare To Zero : simulink/Logic and Bit Operations/Compare To Zero  relop=~=  OutDataTypeStr=boolean
  Compare To Zero1 : simulink/Logic and Bit Operations/Compare To Zero  relop=~=  OutDataTypeStr=boolean
  DSup ends : HitCross  HitCrossingOffset=0.5  HitCrossingDirection=falling  ZeroCross=off
  Data Type Conversion : DataTypeConversion  OutDataTypeStr=double
  Double Support? : Logic  AllPortsSameDT=off
  Double Support?1 : Logic  AllPortsSameDT=off
  Double Support?4 : Logic  AllPortsSameDT=off
  LLeg starts DSup : HitCross  HitCrossingOffset=0.5  HitCrossingDirection=rising  ZeroCross=off
  Memory : Memory
  Memory3 : Memory
  RLeg starts DSup : HitCross  HitCrossingOffset=0.5  HitCrossingDirection=rising  ZeroCross=off
  S-R Flip-Flop : simulink_extras/Flip Flops/S-R Flip-Flop  initial_condition=0
  S-R Flip-Flop1 : simulink_extras/Flip Flops/S-R Flip-Flop  initial_condition=0
  Terminator1 : Terminator
  Terminator2 : Terminator
  RightLeading : Outport
  LeftLeading : Outport  Port=2
  wires:
  S-R Flip-Flop/2 -> Terminator1/1
  S-R Flip-Flop/1 -> LeftLeading/1
  S-R Flip-Flop1/2 -> Terminator2/1
  LStance/1 -> Memory3/1, Compare To Zero/1
  RStance/1 -> Compare To Zero1/1, Memory/1
  S-R Flip-Flop1/1 -> RightLeading/1
  Memory/1 -> RLeg starts DSup/1
  RLeg starts DSup/1 -> Double Support?1/2
  Double Support?1/1 -> S-R Flip-Flop1/1
  Memory3/1 -> LLeg starts DSup/1
  LLeg starts DSup/1 -> Double Support?4/1
  Double Support?4/1 -> S-R Flip-Flop/1
  DSup ends/1 -> S-R Flip-Flop/2, S-R Flip-Flop1/2
  Compare To Zero/1 -> Double Support?/1
  Compare To Zero1/1 -> Double Support?/2
  Double Support?/1 -> Data Type Conversion/1
  Data Type Conversion/1 -> Double Support?1/1, Double Support?4/2, DSup ends/1

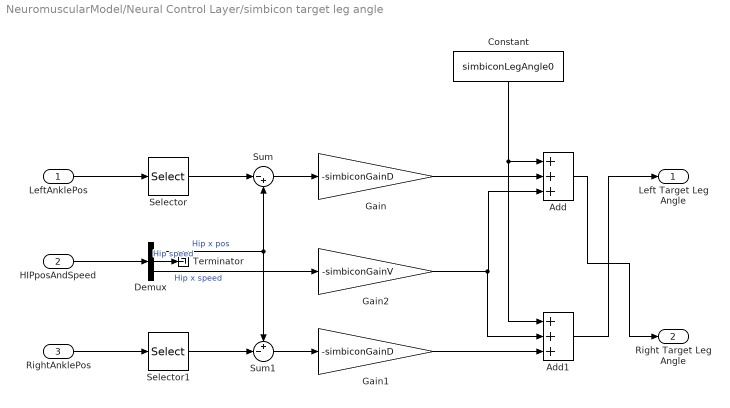
== system NeuromuscularModel/Neural Control Layer/simbicon target leg angle ==
  LeftAnklePos : Inport
  HIPposAndSpeed : Inport  Port=2
  RightAnklePos : Inport  Port=3
  Add : Sum  Inputs=+++
  Add1 : Sum  Inputs=+++
  Constant : Constant  Value=simbiconLegAngle0
  Demux : Demux  Outputs=3
  Gain : Gain  Gain=-simbiconGainD
  Gain1 : Gain  Gain=-simbiconGainD
  Gain2 : Gain  Gain=-simbiconGainV
  Selector : Selector  InputPortWidth=3  IndexOptions=Index vector (dialog)  Indices=[1]  OutputSizes=1
  Selector1 : Selector  InputPortWidth=3  IndexOptions=Index vector (dialog)  Indices=[1]  OutputSizes=1
  Sum : Sum  Inputs=|-+
  Sum1 : Sum  Inputs=+-|
  Terminator : Terminator
  Left Target Leg Angle : Outport
  Right Target Leg Angle : Outport  Port=2
  wires:
  HIPposAndSpeed/1 -> Demux/1
  Demux/1 -> Sum/2, Sum1/1  "Hip x pos"
  Sum/1 -> Gain/1
  Sum1/1 -> Gain1/1
  Gain/1 -> Add/2
  Gain2/1 -> Add1/2, Add/3
  Gain1/1 -> Add1/3
  Constant/1 -> Add/1, Add1/1
  Add1/1 -> Left Target Leg Angle/1
  Add/1 -> Right Target Leg Angle/1
  LeftAnklePos/1 -> Selector/1
  Selector/1 -> Sum/1
  RightAnklePos/1 -> Selector1/1
  Selector1/1 -> Sum1/2
  Demux/3 -> Gain2/1  "Hip x speed"
  Demux/2 -> Terminator/1  "Hip speed"
